simulink model "power_kundur_statcom01"  (R2021a)
settings: Solver=ode23tb  StartTime=0.0  StopTime=10  MaxStep=1/60  RelTol=1e-4  EnableMultiTasking=on
values from neighbouring files (symbols this model uses):
  j = 1    [OABC_PSO_TUNED_NOFault.mat]    (also in OABC_PSO_TUNED_ThreePHASEFault.mat; Traditional_ABC_PSO2.m = randi([1 noFood], 1))
  kk = [0 0.302628193662]    [OABC_PSO_TUNED_NOFault.mat]    (also in OABC_PSO_TUNED_ThreePHASEFault.mat = [6.69502367045 1584.585174])
undefined symbols (not defined in the file or in its folder): Ac, Bc, Cc, D1, Dc, Delta, Fnom, gcbh, K_Vdq2m_SH, Kf_I_SH, Ki_I_SH, Ki_Vac_SH, Ki_Vdc_SH, Kp_I_SH, Kp_Vac_SH, Kp_Vdc_SH, L_RL_SH, MagIinit_SH, PhaIinit_SH, R_RL_SH, sps_rtmsupport, VdcRef_SH, Vnom_SH, xfo_ratio_SH
libraries: spsGenericPowerSystemStabilizerLib x8, spsLoadFlowBusLib x6, spsThreePhaseParallelRLCLoadLib x4, spsThreePhasePISectionLineLib x4, spsSynchronousMachinepuStandardLib x4, spsExcitationSystemLib x4, spsMultiBandPowerSystemStabilizerLib x4, spsSteamTurbineandGovernorLib x4, spsThreePhaseTransformerTwoWindingsLib x4, spsThreePhaseVIMeasurementLib x3, spsThreePhaseBreakerLib x2, spsControlledCurrentSourceLib x2
(part 3 of 3)

== system power_kundur_statcom01/100 MVA STATCOM1/statcom_control/Current Regulator/PI ==
  In1 : Inport
  -1<Id<+1 : Saturate  UpperLimit=UpperLimit  LowerLimit=LowerLimit
  Integrator : Integrator  InitialCondition=Init  LimitOutput=on  UpperSaturationLimit=UpperLimit  LowerSaturationLimit=LowerLimit  AbsoluteTolerance=1e-5
  Kp4 : Gain  Gain=Kp_I  SaturateOnIntegerOverflow=on  OutDataTypeStr=Inherit: Same as input  ParamDataTypeStr=Inherit: Same as input
  Kp5 : Gain  Gain=Ki_I  SaturateOnIntegerOverflow=on  OutDataTypeStr=Inherit: Same as input  ParamDataTypeStr=Inherit: Same as input
  Sum6 : Sum  InputSameDT=on  SaturateOnIntegerOverflow=on  OutDataTypeStr=Inherit: Same as first input
  Out1 : Outport  VectorParamsAs1DForOutWhenUnconnected=off
  wires:
  -1<Id<+1/1 -> Out1/1
  Sum6/1 -> -1<Id<+1/1
  In1/1 -> Kp4/1, Kp5/1
  Integrator/1 -> Sum6/2
  Kp4/1 -> Sum6/1
  Kp5/1 -> Integrator/1

== system power_kundur_statcom01/100 MVA STATCOM1/statcom_control/Current Regulator/PI1 ==
  In1 : Inport
  -1<Id<+1 : Saturate  UpperLimit=UpperLimit  LowerLimit=LowerLimit
  Integrator : Integrator  InitialCondition=Init  LimitOutput=on  UpperSaturationLimit=UpperLimit  LowerSaturationLimit=LowerLimit  AbsoluteTolerance=1e-5
  Kp4 : Gain  Gain=Kp_I  SaturateOnIntegerOverflow=on  OutDataTypeStr=Inherit: Same as input  ParamDataTypeStr=Inherit: Same as input
  Kp5 : Gain  Gain=Ki_I  SaturateOnIntegerOverflow=on  OutDataTypeStr=Inherit: Same as input  ParamDataTypeStr=Inherit: Same as input
  Sum6 : Sum  InputSameDT=on  SaturateOnIntegerOverflow=on  OutDataTypeStr=Inherit: Same as first input
  Out1 : Outport  VectorParamsAs1DForOutWhenUnconnected=off
  wires:
  Kp5/1 -> Integrator/1
  Kp4/1 -> Sum6/1
  Integrator/1 -> Sum6/2
  In1/1 -> Kp5/1, Kp4/1
  Sum6/1 -> -1<Id<+1/1
  -1<Id<+1/1 -> Out1/1

== system power_kundur_statcom01/100 MVA STATCOM1/Power Components Modeling (Shunt & Series Converter)/Power Components modeling (Shunt Converter)/dq-axis model of 3-ph RL branch/Positive-sequence d-q axis model of a 3-phase series R-L branch ==
  note: where w = 2*pi*Fnom (Hz)
  note: Vq1 - Vq2 = [ R * Iq ] + [ L* w * Id ] + [ L * d/dt (Iq) ]
  note: ==========================================================================================
  note: I --->
  note: V2
  note: V1
  note: o--------| R |---| L |-------o
  note: Vd1 - Vd2 = [ R * Id ] - [ L* w * Iq ] + [ L * d/dt (Id) ]
  note: where w = 2*pi*Fnom (Hz)
  note: Iq = [ w / ( L * s ) ] * [ Vq1 - Vq2 - ( R * Iq ) - ( L * Id ) ]
  note: Id = [ w / ( L * s ) ] * [ Vd1 - Vd2 - ( R * Id ) + ( L * Iq ) ]
  note: d-q axis model of a 3-phase series R-L branch
  note: Using Laplace transform and per unit (pu) quantities :
  Vdq1 : Inport
  Vdq2 : Inport  Port=2
  R_RL : Inport  Port=3
  Integrator : Integrator  InitialCondition="[MagIinit_SH*cos(PhaIinit_SH*pi/180)  MagIinit_SH*sin(PhaIinit_SH*pi/180)]"
  Product : Product  SaturateOnIntegerOverflow=on  OutDataTypeStr=Inherit: Same as first input
  R_choke1 : Gain  Gain=L  SaturateOnIntegerOverflow=on  OutDataTypeStr=Inherit: Same as input  ParamDataTypeStr=Inherit: Same as input
  R_choke2 : Gain  Gain=[1 -1]  SaturateOnIntegerOverflow=on  OutDataTypeStr=Inherit: Same as input  ParamDataTypeStr=Inherit: Same as input
  R_choke3 : Gain  Gain=w / L  SaturateOnIntegerOverflow=on  OutDataTypeStr=Inherit: Same as input  ParamDataTypeStr=Inherit: Same as input
  Selector : Selector  InputPortWidth=2  IndexOptions=Index vector (dialog)  Indices=[2 1]  OutputSizes=1
  Sum : Sum  Inputs=+--+  SaturateOnIntegerOverflow=on
  idIq : Outport  VectorParamsAs1DForOutWhenUnconnected=off
  wires:
  Selector/1 -> R_choke1/1
  Integrator/1 -> Selector/1, Product/2, idIq/1
  R_choke3/1 -> Integrator/1
  Sum/1 -> R_choke3/1
  R_choke1/1 -> R_choke2/1
  R_choke2/1 -> Sum/4
  Product/1 -> Sum/3
  Vdq2/1 -> Sum/2
  Vdq1/1 -> Sum/1
  R_RL/1 -> Product/1

== system power_kundur_statcom01/100 MVA STATCOM1/Power Components Modeling (Shunt & Series Converter)/Power Components modeling (Shunt Converter)/dq-axis model of 3-ph RL branch/abc2dq ==
  note: V1= 1/3(Va +aVb+a^2*Vc)
  note: where a=exp(2*pi/3*j)
  Vabc cmplx : Inport
  Complex to Real-Imag : ComplexToRealImag
  Demux : Demux  Outputs=3
      settings: DisplayOption=none
  Gain2 : Gain  Gain=1/3  SaturateOnIntegerOverflow=on  OutDataTypeStr=Inherit: Same as input  ParamDataTypeStr=Inherit: Same as input
  Mux : Mux  Inputs=2
  Sum3 : Sum  Inputs=+++  InputSameDT=on  SaturateOnIntegerOverflow=on  OutDataTypeStr=Inherit: Same as first input
  a : Gain  Gain=exp(j*2*pi/3)  SaturateOnIntegerOverflow=on  OutDataTypeStr=Inherit: Same as input  ParamDataTypeStr=Inherit: Same as input
  a^2 : Gain  Gain=exp(-j*2*pi/3)  SaturateOnIntegerOverflow=on  OutDataTypeStr=Inherit: Same as input  ParamDataTypeStr=Inherit: Same as input
  Vdq_seq1 : Outport  VectorParamsAs1DForOutWhenUnconnected=off
  wires:
  Vabc cmplx/1 -> Demux/1
  Sum3/1 -> Gain2/1  "V1"
  Demux/1 -> Sum3/1
  a/1 -> Sum3/2
  a^2/1 -> Sum3/3
  Complex to Real-Imag/1 -> Mux/1
  Complex to Real-Imag/2 -> Mux/2
  Demux/2 -> a/1
  Demux/3 -> a^2/1
  Mux/1 -> Vdq_seq1/1
  Gain2/1 -> Complex to Real-Imag/1

== system power_kundur_statcom01/100 MVA STATCOM1/Power Components Modeling (Shunt & Series Converter)/Power Components modeling (Shunt Converter)/dq-axis model of 3-ph RL branch/abc2dq1 ==
  note: where a=exp(2*pi/3*j)
  note: V1= 1/3(Va +aVb+a^2*Vc)
  Vabc cmplx : Inport
  Complex to Real-Imag : ComplexToRealImag
  Demux : Demux  Outputs=3
      settings: DisplayOption=none
  Gain2 : Gain  Gain=1/3  SaturateOnIntegerOverflow=on  OutDataTypeStr=Inherit: Same as input  ParamDataTypeStr=Inherit: Same as input
  Mux : Mux  Inputs=2
  Sum3 : Sum  Inputs=+++  InputSameDT=on  SaturateOnIntegerOverflow=on  OutDataTypeStr=Inherit: Same as first input
  a : Gain  Gain=exp(j*2*pi/3)  SaturateOnIntegerOverflow=on  OutDataTypeStr=Inherit: Same as input  ParamDataTypeStr=Inherit: Same as input
  a^2 : Gain  Gain=exp(-j*2*pi/3)  SaturateOnIntegerOverflow=on  OutDataTypeStr=Inherit: Same as input  ParamDataTypeStr=Inherit: Same as input
  Vdq_seq1 : Outport  VectorParamsAs1DForOutWhenUnconnected=off
  wires:
  Gain2/1 -> Complex to Real-Imag/1
  Mux/1 -> Vdq_seq1/1
  Demux/3 -> a^2/1
  Demux/2 -> a/1
  Complex to Real-Imag/2 -> Mux/2
  Complex to Real-Imag/1 -> Mux/1
  a^2/1 -> Sum3/3
  a/1 -> Sum3/2
  Demux/1 -> Sum3/1
  Sum3/1 -> Gain2/1  "V1"
  Vabc cmplx/1 -> Demux/1

== system power_kundur_statcom01/100 MVA STATCOM1/Power Components Modeling (Shunt & Series Converter)/Power Components modeling (Shunt Converter)/dq-axis model of 3-ph RL branch/dq2ab ==
  note: Ia = I1
      | Ib = (a^2 * I1)
  Idq_seq1 : Inport
  Demux1 : Demux  Outputs=2
      settings: DisplayOption=none
  Mux : Mux  Inputs=2
  Real-Imag to Complex1 : RealImagToComplex
  a^2 : Gain  Gain=exp(-j*2*pi/3)  SaturateOnIntegerOverflow=on  OutDataTypeStr=Inherit: Same as input  ParamDataTypeStr=Inherit: Same as input
  Ia_Ib complx : Outport  VectorParamsAs1DForOutWhenUnconnected=off
  wires:
  Mux/1 -> Ia_Ib complx/1
  Idq_seq1/1 -> Demux1/1
  Demux1/1 -> Real-Imag to Complex1/1
  Demux1/2 -> Real-Imag to Complex1/2
  Real-Imag to Complex1/1 -> Mux/1, a^2/1  "I1"
  a^2/1 -> Mux/2
